simulink model "PI_Control"  (R2018b)
settings: Solver=VariableStepAuto  StartTime=0.0  StopTime=300  MaxStep=0.5  RelTol=1e-3
libraries: simulink x2
settings Model: Creator=ian  LastModifiedBy=Vishant
settings SFSimCC: SimUseLocalCustomCode=off
settings RTWCC: RTWUseLocalCustomCode=off
settings CodeAppCC: StateflowObjectComments=on

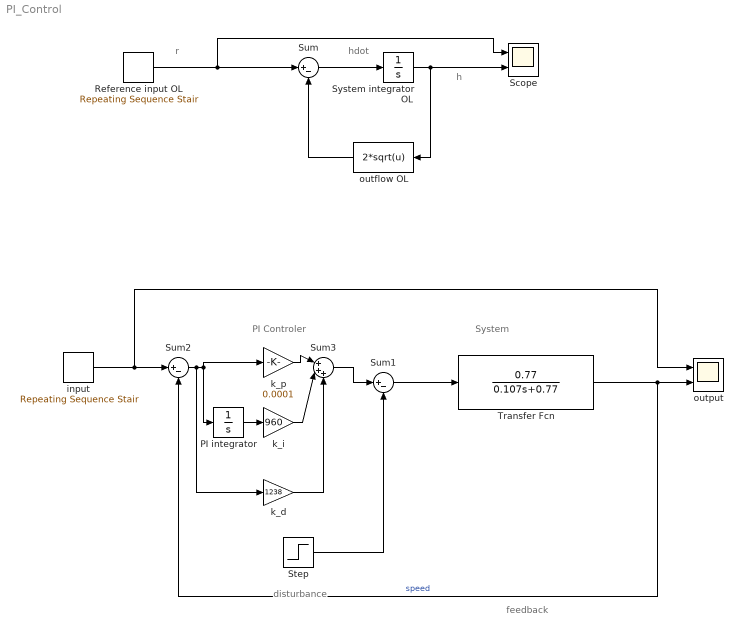
== system PI_Control ==
  note: disturbance
  note: feedback
  note: System
  note: PI Controler
  note: hdot
  note: h
  note: r
  PI integrator : Integrator  InitialCondition=3
  Reference input OL : simulink/Sources/Repeating Sequence Stair  OutValues=[5 2 6 4 1 3].'  tsamp=50  OutMin=[]  OutMax=[]  OutDataTypeStr=double  OutputDataTypeScalingMode=double  OutDataType=fixdt(0,8)  ConRadixGroup=Best Precision: Vector-wise  OutScaling=2^-12
  Scope : Scope  NumInputPorts=2
  Step : Step  After=2383.73  SampleTime=0
  Sum : Sum  Inputs=|+-
  Sum1 : Sum  Inputs=|+-
  Sum2 : Sum  Inputs=|+-
  Sum3 : Sum  Inputs=|+++
  System integrator OL : Integrator  InitialCondition=3
  Transfer Fcn : TransferFcn  Numerator=[0.77]  Denominator=[0.107 0.77]
  input : simulink/Sources/Repeating Sequence Stair  OutValues=[-10].'  tsamp=50  OutMin=[]  OutMax=[]  OutDataTypeStr=double  OutputDataTypeScalingMode=double  OutDataType=fixdt(0,8)  ConRadixGroup=Best Precision: Vector-wise  OutScaling=2^-12
  k_d : Gain  Gain=1238
  k_i : Gain  Gain=960
  k_p : Gain  Gain=0.0001
  outflow OL : Fcn  Expr=2*sqrt(u)
  output : Scope  NumInputPorts=2
  wires:
  Sum/1 -> System integrator OL/1
  outflow OL/1 -> Sum/2
  System integrator OL/1 -> Scope/2, outflow OL/1
  Reference input OL/1 -> Scope/1, Sum/1
  input/1 -> output/1, Sum2/1
  Sum3/1 -> Sum1/1
  PI integrator/1 -> k_i/1
  Sum2/1 -> PI integrator/1, k_p/1, k_d/1
  k_p/1 -> Sum3/1
  k_i/1 -> Sum3/2
  Step/1 -> Sum1/2
  Sum1/1 -> Transfer Fcn/1
  Transfer Fcn/1 -> output/2, Sum2/2  "speed"
  k_d/1 -> Sum3/3
